simulink model "segmentCalcNeg"  (R2019a)
settings: Solver=VariableStepAuto  StartTime=0  StopTime=inf  FixedStep=1/100  MaxStep=1e-3  RelTol=1e-3
values from neighbouring files (symbols this model uses):
  apexVelocity = apexData.velocity(n,2)    [calcSegments.m]
  course = addRadius(course,max(vRLookUp(:,1)))    [calcggV.m]    (also in importCourse.m = addRadius(course))
  currentDistance = apexData.locs(n,1) - 1    [calcSegments.m]
  stoppingDistance = apexData.locs(n+1,1) - 1    [calcSegments.m]
undefined symbols (not defined in the file or in its folder): init
libraries: simulink x1
settings Model: Creator=Frieder Uerlings  LastModifiedBy=Frieder Uerlings

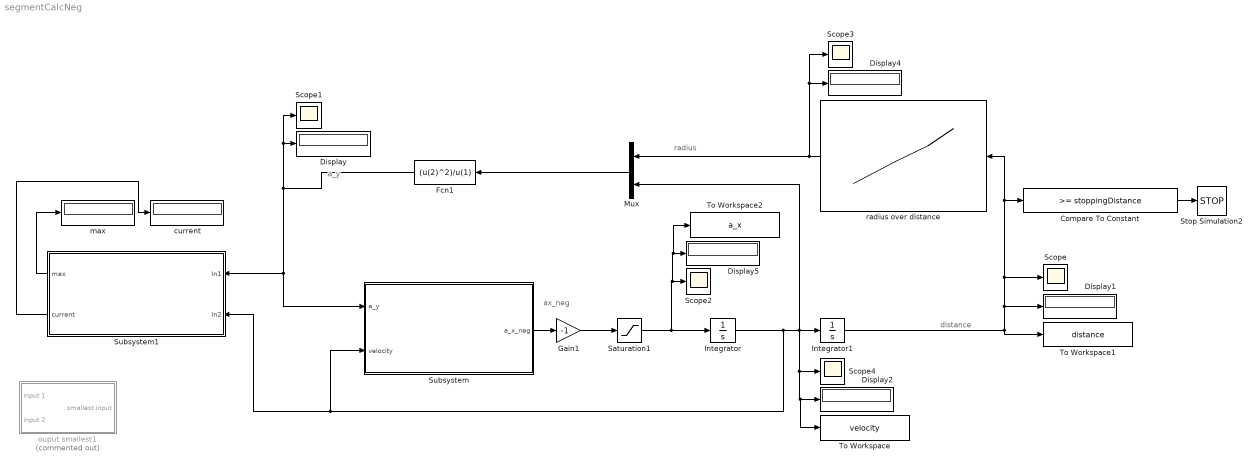
== system segmentCalcNeg ==
  note: a_y
  note: radius
  note: distance
  note: ax_neg
  Compare To Constant : simulink/Logic and Bit Operations/Compare To Constant  relop=>=  const=stoppingDistance  OutDataTypeStr=boolean
  Display{,1..2,4..5} (5 alike) : Display
  Fcn1 : Fcn  Expr=(u(2)^2)/u(1)
  Gain1 : Gain  Gain=-1
  Integrator : Integrator  InitialCondition=apexVelocity
  Integrator1 : Integrator  InitialCondition=currentDistance
  Mux : Mux  Inputs=2
  Saturation1 : Saturate  UpperLimit=inf  LowerLimit=0
  Scope{,1..4} (5 alike) : Scope
  Stop Simulation2 : Stop
  Subsystem : Subsystem
  Subsystem1 : Subsystem
  To Workspace : ToWorkspace  VariableName=velocity  SampleTime=-1
  To Workspace1 : ToWorkspace  VariableName=distance  SampleTime=-1
  To Workspace2 : ToWorkspace  VariableName=a_x  SampleTime=-1
  current : Display
  "max " : Display
  ouput smallest1 : Subsystem  Commented=on
  radius over distance : Lookup_n-D  NumberOfTableDimensions=1  BreakpointsForDimension1=[0:1:length(course)-1]  Table=flip(course(:,3))  InternalRulePriority=Speed  RndMeth=Simplest  InputSameDT=on
  wires:
  radius over distance/1 -> Mux/1, Scope3/1, Display4/1
  Mux/1 -> Fcn1/1
  Subsystem/1(a_x_neg) -> Gain1/1
  Fcn1/1 -> Subsystem/1("a_y "), Subsystem1/1(In1), Display/1, Scope1/1
  Subsystem1/1("max ") -> "max "/1
  Subsystem1/2("current ") -> current/1
  Integrator/1 -> Mux/2, To Workspace/1, Display2/1, Scope4/1, Integrator1/1, Subsystem/2("velocity "), Subsystem1/2(In2)
  Compare To Constant/1 -> Stop Simulation2/1
  Integrator1/1 -> To Workspace1/1, Scope/1, Compare To Constant/1, radius over distance/1, Display1/1
  Gain1/1 -> Saturation1/1
  Saturation1/1 -> To Workspace2/1, Display5/1, Scope2/1, Integrator/1

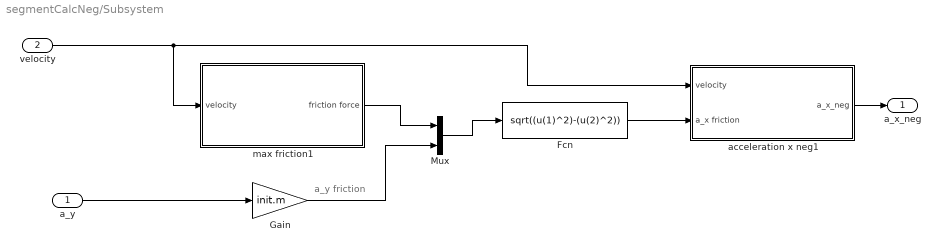
== system segmentCalcNeg/Subsystem ==
  note: a_y friction
  "a_y " : Inport
  "velocity " : Inport  Port=2
  Fcn : Fcn  Expr=sqrt((u(1)^2)-(u(2)^2))
  Gain : Gain  Gain=init.m
  Mux : Mux  Inputs=2
  acceleration x neg1 : Subsystem
  max friction1 : Subsystem
  a_x_neg : Outport
  wires:
  "velocity "/1 -> max friction1/1(velocity), acceleration x neg1/1(velocity)
  "a_y "/1 -> Gain/1
  Fcn/1 -> acceleration x neg1/2(a_x friction)
  Mux/1 -> Fcn/1
  acceleration x neg1/1("a_x_neg ") -> a_x_neg/1
  max friction1/1(friction force) -> Mux/1
  Gain/1 -> Mux/2

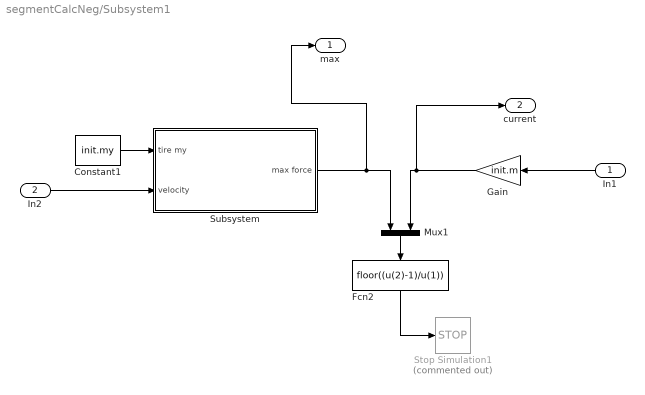
== system segmentCalcNeg/Subsystem1 ==
  In1 : Inport
  In2 : Inport  Port=2
  Constant1 : Constant  Value=init.my
  Fcn2 : Fcn  Expr=floor((u(2)-1)/u(1))
  Gain : Gain  Gain=init.m
  Mux1 : Mux  Inputs=2
  Stop Simulation1 : Stop  Commented=on
  Subsystem : Subsystem
  "max " : Outport
  "current " : Outport  Port=2
  wires:
  Gain/1 -> "current "/1, Mux1/2
  Fcn2/1 -> Stop Simulation1/1
  Mux1/1 -> Fcn2/1
  Constant1/1 -> Subsystem/1(tire my)
  In1/1 -> Gain/1
  Subsystem/1(max force) -> "max "/1, Mux1/1
  In2/1 -> Subsystem/2(velocity)

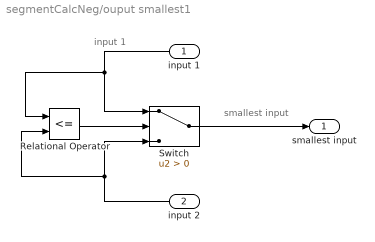
== system segmentCalcNeg/ouput smallest1 ==
  note: input 1
  note: smallest input
  "input 1 " : Inport
  "input 2 " : Inport  Port=2
  Relational Operator : RelationalOperator  Operator=<=  OutDataTypeStr=boolean  RndMeth=Simplest
  Switch : Switch  Criteria=u2 > Threshold
  smallest input : Outport
  wires:
  Relational Operator/1 -> Switch/2
  Switch/1 -> smallest input/1
  "input 1 "/1 -> Switch/1, Relational Operator/1
  "input 2 "/1 -> Switch/3, Relational Operator/2

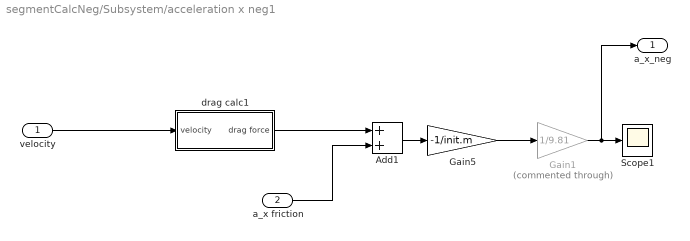
== system segmentCalcNeg/Subsystem/acceleration x neg1 ==
  velocity : Inport
  a_x friction : Inport  Port=2
  Add1 : Sum
  Gain1 : Gain  Commented=through  Gain=1/9.81
  Gain5 : Gain  Gain=-1/init.m
  Scope1 : Scope
  drag calc1 : Subsystem
  "a_x_neg " : Outport
  wires:
  drag calc1/1("drag force ") -> Add1/1
  a_x friction/1 -> Add1/2
  velocity/1 -> drag calc1/1(velocity)
  Gain1/1 -> "a_x_neg "/1, Scope1/1
  Add1/1 -> Gain5/1
  Gain5/1 -> Gain1/1

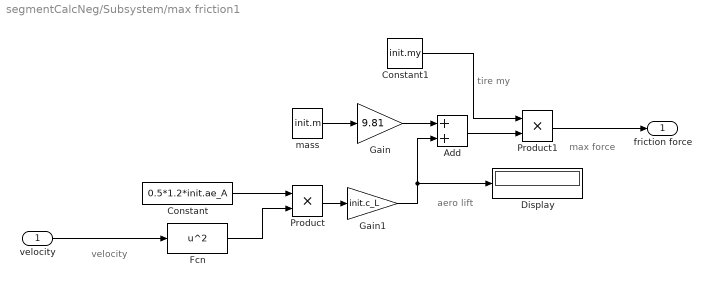
== system segmentCalcNeg/Subsystem/max friction1 ==
  note: velocity
  note: tire my
  note: aero lift
  note: max force
  velocity : Inport
  Add : Sum
  Constant : Constant  Value=0.5*1.2*init.ae_A
  Constant1 : Constant  Value=init.my
  Display : Display
  Fcn : Fcn  Expr=u^2
  Gain : Gain  Gain=9.81
  Gain1 : Gain  Gain=init.c_L
  Product : Product
  Product1 : Product
  "mass " : Constant  Value=init.m
  friction force : Outport
  wires:
  Gain1/1 -> Display/1, Add/2
  velocity/1 -> Fcn/1
  Constant1/1 -> Product1/1
  Product/1 -> Gain1/1
  Gain/1 -> Add/1
  Product1/1 -> friction force/1
  Fcn/1 -> Product/2
  "mass "/1 -> Gain/1
  Add/1 -> Product1/2
  Constant/1 -> Product/1

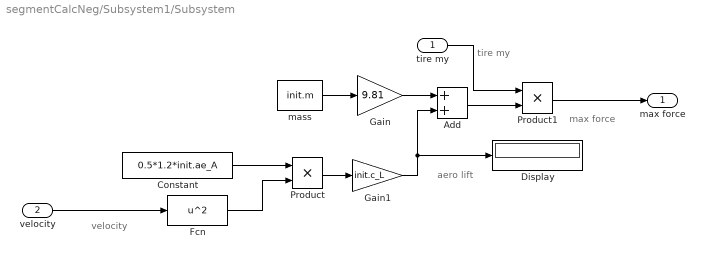
== system segmentCalcNeg/Subsystem1/Subsystem ==
  note: max force
  note: aero lift
  note: tire my
  note: velocity
  tire my : Inport
  velocity : Inport  Port=2
  Add : Sum
  Constant : Constant  Value=0.5*1.2*init.ae_A
  Display : Display
  Fcn : Fcn  Expr=u^2
  Gain : Gain  Gain=9.81
  Gain1 : Gain  Gain=init.c_L
  Product : Product
  Product1 : Product
  "mass " : Constant  Value=init.m
  max force : Outport
  wires:
  Constant/1 -> Product/1
  Add/1 -> Product1/2
  "mass "/1 -> Gain/1
  Fcn/1 -> Product/2
  Product1/1 -> max force/1
  Gain/1 -> Add/1
  Product/1 -> Gain1/1
  tire my/1 -> Product1/1
  velocity/1 -> Fcn/1
  Gain1/1 -> Add/2, Display/1

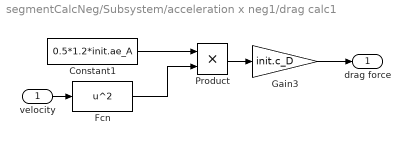
== system segmentCalcNeg/Subsystem/acceleration x neg1/drag calc1 ==
  velocity : Inport
  Constant1 : Constant  Value=0.5*1.2*init.ae_A
  Fcn : Fcn  Expr=u^2
  Gain3 : Gain  Gain=init.c_D
  Product : Product
  "drag force " : Outport
  wires:
  Constant1/1 -> Product/1
  velocity/1 -> Fcn/1
  Fcn/1 -> Product/2
  Product/1 -> Gain3/1
  Gain3/1 -> "drag force "/1
